simulink model "sim_7_on_off_button"  (R2022b)
settings: Solver=VariableStepAuto  StartTime=0.0  StopTime=inf  RelTol=1e-3
settings Model: Creator=user  LastModifiedBy=user

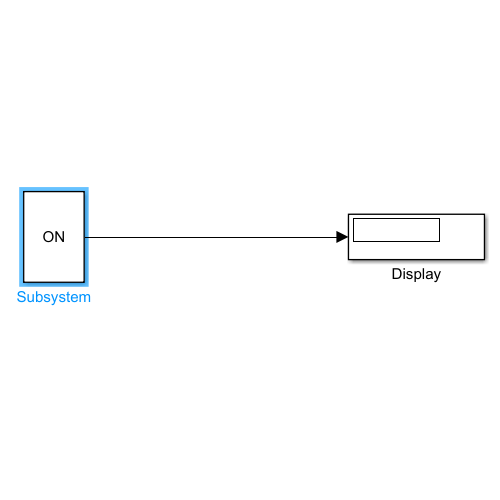
[thumbnail: Simulink's stored preview of the top-level diagram]
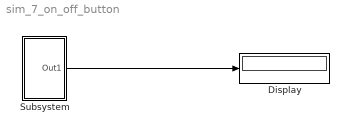
== system sim_7_on_off_button ==
  Display : Display
  Subsystem : Subsystem  StartFcn=|  mask{str=ON}
      | set_param(gcb, 'str', 'OFF');
      | set_param([gcb,'/C'], 'Value', '0');
      mask prompts: str "Display Name :"
      settings: OpenFcn=|
      | old_val = get_param([gcb, '/C'], 'Value');
      | 
      | switch old_val
      |  case '0'
      |   set_param(gcb, 'str', 'ON');
      |   set_param([gcb, '/C'], 'Value', '1');
      |  case '1'
      |   set_param(gcb, 'str', 'OFF');
      |   set_param([gcb,'/C'], 'Value', '0');
      |  otherwise
      |   set_param(gcb, 'str', 'OFF');
      |   set_param([gcb,'/C'], 'Value', '0');
      | end
      mask DialogControl ParameterGroupVar Prompt: 파라미터
      mask Display:
      | blk_name = get_param(gcb, 'str');
      | disp(blk_name);
  wires:
  Subsystem/1(Out1) -> Display/1

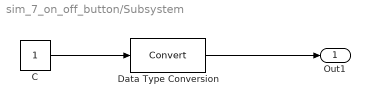
== system sim_7_on_off_button/Subsystem ==
  C : Constant
  Data Type Conversion : DataTypeConversion  SaturateOnIntegerOverflow=off  RndMeth=Floor
  Out1 : Outport
  wires:
  C/1 -> Data Type Conversion/1
  Data Type Conversion/1 -> Out1/1
